simulink library "library_mtu_simulink"  (R2019a)
settings: Solver=VariableStepAuto  StartTime=0.0  StopTime=10.0  RelTol=1e-3  EnableMultiTasking=on
values from neighbouring files (symbols this model uses):
  MP = muscle_param_GM_exp    [init_muscle_exp.m]
undefined symbols (not defined in the file or in its folder): stim0
libraries: $bdroot x3
settings Model: Creator=danielhaeufle  LastModifiedBy=danielhaeufle
settings DataIOCC: LimitDataPoints=on  ReturnWorkspaceOutputs=off
settings OptimizationCC: LifeSpan=inf
settings DebuggingCC: AllowSymbolicDim=off  PregeneratedLibrarySubsystemCodeDiagnostic=none  SFUnexpectedBacktrackingDiag=warning  SFNoUnconditionalDefaultTransitionDiag=warning  SFExecutionAtInitializationDiag=none  ArithmeticOperatorsInVariantConditions=warning
settings ModelReferenceCC: PropagateSignalLabelsOutOfModel=off
settings SFSimCC: SimUseLocalCustomCode=off
settings RTWCC: RTWUseLocalCustomCode=off
settings CodeAppCC: StateflowObjectComments=on
settings GRTTargetCC: TargetLangStandard=C89/C90 (ANSI)
settings ConfigComp: CovMetricSettings=dw  CovHtmlReporting=on  CovSaveCumulativeToWorkspaceVar=on  CovSaveSingleToWorkspaceVar=on  CovExternalEMLEnable=off

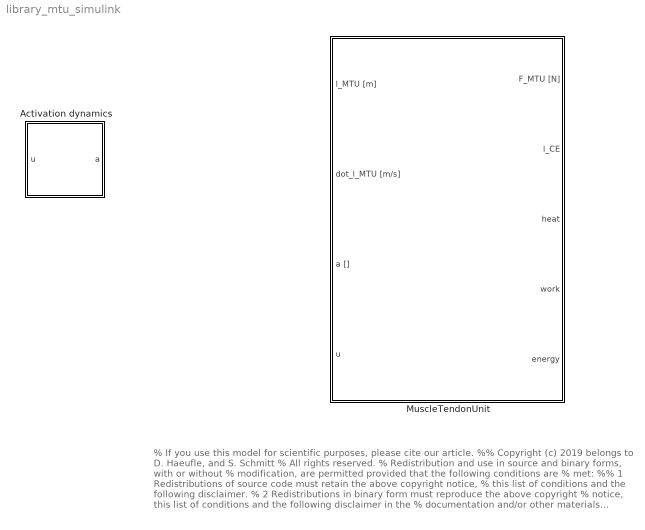
== system library_mtu_simulink ==
  note: % If you use this model for scientific purposes, please cite our article.
      | %% Copyright (c) 2019 belongs to D. Haeufle, and S. Schmitt % All rights reserved.
      | % Redistribution and use in source and binary forms, with or without
      | % modification, are permitted provided that the following conditions are
      | % met:
      | %%  1 Redistributions of source code must retain the above copyright notice,
      | %    this list of conditions and the following disclaimer.
      | %  2 Redistributions in binary form must reproduce the above copyright
      | %    notice, this list of conditions and the following disclaimer in the
      | %    documentation and/or other materials provided with the distribution.
      | %  3 Neither the name of the owner nor the names of its contributors may be
      | %    used to endorse or promote products derived from this software without
      | %    specific prior written permission.
      | %% THIS SOFTWARE IS PROVIDED BY THE COPYRIGHT HOLDERS AND CONTRIBUTORS "AS
      | % IS" AND ANY EXPRESS OR IMPLIED WARRANTIES, INCLUDING, BUT NOT LIMITED TO,
      | % THE IMPLIED WARRANTIES OF MERCHANTABILITY AND FITNESS FOR A PARTICULAR
      | % PURPOSE ARE DISCLAIMED. IN NO EVENT SHALL THE COPYRIGHT HOLDER BE LIABLE
      | % FOR ANY DIRECT, INDIRECT, INCIDENTAL, SPECIAL, EXEMPLARY, OR
      | % CONSEQUENTIAL DAMAGES (INCLUDING, BUT NOT LIMITED TO, PROCUREMENT OF
      | % SUBSTITUTE GOODS OR SERVICES; LOSS OF USE, DATA, OR PROFITS; OR BUSINESS
      | % INTERRUPTION) HOWEVER CAUSED AND ON ANY THEORY OF LIABILITY, WHETHER IN
      | % CONTRACT, STRICT LIABILITY, OR TORT (INCLUDING NEGLIGENCE OR OTHERWISE)
      | % ARISING IN ANY WAY OUT OF THE USE OF THIS SOFTWARE, EVEN IF ADVISED OF
      | % THE POSSIBILITY OF SUCH DAMAGE.
  Activation dynamics : Subsystem  mask{Mus_Param=MP(1)}
      mask prompts: Mus_Param "Muscle parameter struct"
  MuscleTendonUnit : Subsystem  mask(Muscle Tendon Complex Model){Mus_Param=MP(1)}
      mask prompts: Mus_Param "Muscle parameter struct"
      mask help: This block returns the muscle tendon complex (MTC) force based on muscle length l_MTC, contraction velocity dot_l_MTC, and activity q
      mask Help:
      | Copyright (c) 2013, D. Haeufle, M. Guenther, A. Bayer, and S. Schmitt
      | All rights reserved.
      | 
      | Redistribution and use in source and binary forms, with or without modification, are permitted provided that the following conditions are met:
      | 
      |     Redistributions of source code must retain the above copyright notice, this list of conditions and the following disclaimer.
      |     Redistributions in binary form must reproduce the above copyright notice, this list of conditions and the following disclaimer in the documentation and/or other materials provided with the distribution.
      |     Neither the name of the <ORGANIZATION> nor the names of its contributors may be used to endorse or promote products derived from this software without specific prior written permission.
      | 
      | THIS SOFTWARE IS PROVIDED BY THE COPYRIGHT HOLDERS AND CONTRIBUTORS "AS IS" AND ANY EXPRESS OR IMPLIED WARRANTIES, INCLUDING, BUT NOT LIMITED TO, THE IMPLIED WARRANTIES OF MERCHANTABILITY AND FITNESS FOR A PARTICULAR PURPOSE ARE DISCLAIMED. IN NO EVENT SHALL THE COPYRIGHT HOLDER OR CONTRIBUTORS BE LIABLE FOR ANY DIRECT, INDIRECT, INCIDENTAL, SPECIAL, EXEMPLARY, OR CONSEQUENTIAL DAMAGES (INCLUDING, BUT NOT LIMITED TO, PROCUREMENT OF SUBSTITUTE GOODS OR SERVICES; LOSS OF USE, DATA, OR PROFITS; OR BUSINESS INTERRUPTION) HOWEVER CAUSED AND ON ANY THEORY OF LIABILITY, WHETHER IN CONTRACT, STRICT LIABILITY, OR TORT (INCLUDING NEGLIGENCE OR OTHERWISE) ARISING IN ANY WAY OUT OF THE USE OF THIS SOFTWARE, EVEN IF ADVISED OF THE POSSIBILITY OF SUCH DAMAGE.
      mask Display: patch([4 4 4 4 3.5 3 2.6 2.2 2 2.2 2.6 3 3.5 4 4 4 4 7 7 7 7 7.5 8 8.4 8.8 9 8.8 8.4 8 7.5 7 7 7 7 4]/20+0.2, [0 2:17 17:-1:2 0 0]/17,[1 0 0])

== system library_mtu_simulink/Activation dynamics ==
  u : Inport
  Add1 : Sum  Inputs=-+
  Add3 : Sum
  Constant : Constant  Value=Mus_Param.act_dyn.c1
  Constant1 : Constant  Value=Mus_Param.act_dyn.c2
  Integrator : Integrator  InitialConditionSource=external  InitialCondition=stim0
  Product : Product
  Product1 : Product
  initial activity : Constant  Value=Mus_Param.a_CE_init
  a : Outport
  wires:
  u/1 -> Product1/1, Add1/2
  Integrator/1 -> Add1/1, a/1
  Product/1 -> Integrator/1
  Add1/1 -> Product/1
  initial activity/1 -> Integrator/2
  Constant/1 -> Product1/2
  Product1/1 -> Add3/1
  Add3/1 -> Product/2
  Constant1/1 -> Add3/2

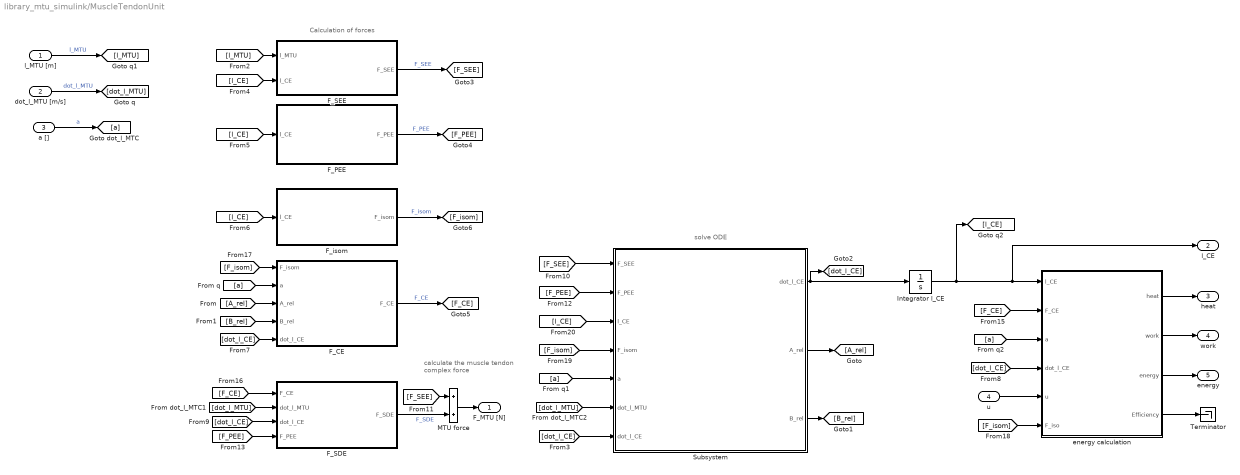
== system library_mtu_simulink/MuscleTendonUnit ==
  note: solve ODE
  note: Calculation of forces
  note: calculate the
      | muscle tendon complex
      | force
  l_MTU [m] : Inport
  dot_l_MTU [m/s] : Inport  Port=2
  a [] : Inport  Port=3
  u : Inport  Port=4
  F_CE : Subsystem
  F_PEE : Subsystem
  F_SDE : Subsystem
  F_SEE : Subsystem
  F_isom : Subsystem
  Integrator l_CE : Integrator  InitialCondition=Mus_Param.l_CE_init  ZeroCross=off
  MTU force : Sum
  Subsystem : Subsystem
  Terminator : Terminator
  energy calculation : Subsystem
  F_MTU [N] : Outport
  l_CE : Outport  Port=2
  heat : Outport  Port=3
  work : Outport  Port=4
  energy : Outport  Port=5
  wires:
  F_isom/1(F_isom) -> [F_isom]  "F_isom"
  F_PEE/1(F_PEE) -> [F_PEE]  "F_PEE"
  F_SEE/1(F_SEE) -> [F_SEE]  "F_SEE"
  F_CE/1(F_CE) -> [F_CE]  "F_CE"
  F_SDE/1(F_SDE) -> MTU force/2  "F_SDE"
  MTU force/1 -> F_MTU [N]/1
  [a] -> F_CE/2(a)
  [a] -> Subsystem/5("a ")
  [dot_l_CE] -> Subsystem/7(dot_l_CE)
  [dot_l_MTU] -> F_SDE/2(dot_l_MTU)
  Subsystem/2(A_rel) -> [A_rel]
  a []/1 -> [a]  "a"
  energy calculation/1(heat) -> heat/1
  u/1 -> energy calculation/5(u)
  energy calculation/2(work) -> work/1
  [A_rel] -> F_CE/3(A_rel)
  [B_rel] -> F_CE/4(B_rel)
  Subsystem/3(B_rel) -> [B_rel]
  Integrator l_CE/1 -> [l_CE], l_CE/1, energy calculation/1(l_CE)
  energy calculation/3(energy) -> energy/1
  Subsystem/1("dot_l_CE ") -> [dot_l_CE], Integrator l_CE/1
  l_MTU [m]/1 -> [l_MTU]  "l_MTU"
  dot_l_MTU [m/s]/1 -> [dot_l_MTU]  "dot_l_MTU"
  [l_MTU] -> F_SEE/1(l_MTU)
  [l_CE] -> F_SEE/2(l_CE)
  [l_CE] -> F_PEE/1(l_CE)
  [l_CE] -> F_isom/1(l_CE)
  [dot_l_CE] -> F_CE/5(dot_l_CE)
  [dot_l_CE] -> energy calculation/4(dot_l_CE)
  [a] -> energy calculation/3(a)
  [dot_l_CE] -> F_SDE/3(dot_l_CE)
  [F_SEE] -> Subsystem/1(F_SEE)
  [F_SEE] -> MTU force/1
  [F_PEE] -> Subsystem/2(F_PEE)
  [F_PEE] -> F_SDE/4(F_PEE)
  [F_CE] -> energy calculation/2(F_CE)
  [F_CE] -> F_SDE/1(F_CE)
  [F_isom] -> F_CE/1(F_isom)
  [F_isom] -> energy calculation/6(F_iso)
  [F_isom] -> Subsystem/4(F_isom)
  [l_CE] -> Subsystem/3(l_CE)
  [dot_l_MTU] -> Subsystem/6(dot_l_MTU)
  energy calculation/4(Efficiency) -> Terminator/1

== system library_mtu_simulink/MuscleTendonUnit/F_CE ==
  note: force of the contractile element
  F_isom : Inport
  a : Inport  Port=2
  A_rel : Inport  Port=3
  B_rel : Inport  Port=4
  dot_l_CE : Inport  Port=5
  Mux : Mux  Inputs=5
  equation for F_CE : Fcn  Expr="Mus_Param.CE.F_max * (  ( (u(1)*u(4)+u(2)) / ( 1- (u(5)/(u(3)*Mus_Param.CE.l_CEopt)) ) )-u(2) )"
  F_CE : Outport
  wires:
  a/1 -> Mux/1
  A_rel/1 -> Mux/2
  B_rel/1 -> Mux/3
  F_isom/1 -> Mux/4
  dot_l_CE/1 -> Mux/5
  equation for F_CE/1 -> F_CE/1
  Mux/1 -> equation for F_CE/1

== system library_mtu_simulink/MuscleTendonUnit/F_PEE ==
  note: Parallel elastic element force
      |
      | is only calculated if l_CE>PEE slack length
      | to avoid complex numbers with
      | non-integer exponents
  l_CE : Inport
  "F_PEE " : Subsystem
  l_PEE > slack length? : Fcn  Expr=(u>=Mus_Param.PEE.l_PEE0)
  F_PEE : Outport
  wires:
  l_CE/1 -> l_PEE > slack length?/1, "F_PEE "/1(l_PEE)
  "F_PEE "/1(Out1) -> F_PEE/1
  l_PEE > slack length?/1 -> "F_PEE "/Enable

== system library_mtu_simulink/MuscleTendonUnit/F_SDE ==
  note: force of the serial damping element
  F_CE : Inport
  dot_l_MTU : Inport  Port=2
  dot_l_CE : Inport  Port=3
  F_PEE : Inport  Port=4
  Mux : Mux
  equation for F_SDE : Fcn  Expr=Mus_Param.SDE.d_SEmax*((1-Mus_Param.SDE.R_SE)*((u(1)+u(2))/Mus_Param.CE.F_max)+Mus_Param.SDE.R_SE)*(u(3)-u(4))
  F_SDE : Outport
  wires:
  Mux/1 -> equation for F_SDE/1
  F_PEE/1 -> Mux/2
  F_CE/1 -> Mux/1
  equation for F_SDE/1 -> F_SDE/1
  dot_l_MTU/1 -> Mux/3
  dot_l_CE/1 -> Mux/4

== system library_mtu_simulink/MuscleTendonUnit/F_SEE ==
  note: MP.SEE.l_SEEnll = L_SEE (angespannt)
  note: MP.SEE.l_SEE0 = rest length of SEE in [m] (Ruhelage)
  note: Series elastic element force
  l_MTU : Inport
  l_CE : Inport  Port=2
  Add1 : Sum  Inputs=+-
  F_SEE_eq : Subsystem
  F_SEE : Outport
  wires:
  l_CE/1 -> Add1/2
  F_SEE_eq/1(F_SEE) -> F_SEE/1
  Add1/1 -> F_SEE_eq/1(l_SEE)  "l_SE"
  l_MTU/1 -> Add1/1

== system library_mtu_simulink/MuscleTendonUnit/F_isom ==
  note: isometric force-length relation
  l_CE : Inport
  Add : Sum
  ascending branch : Fcn  Expr="(Mus_Param.CE.l_CEopt>u)   *   ( exp( -( abs(  ((u/Mus_Param.CE.l_CEopt)-1)/Mus_Param.CE.DeltaW_limb_asc  ) )^Mus_Param.CE.v_CElimb_asc ) )"
  descending branch : Fcn  Expr="(Mus_Param.CE.l_CEopt<=u)   *   ( exp( -( abs(  ((u/Mus_Param.CE.l_CEopt)-1)/Mus_Param.CE.DeltaW_limb_des  ) )^Mus_Param.CE.v_CElimb_des ) )"
  F_isom : Outport
  wires:
  l_CE/1 -> descending branch/1, ascending branch/1
  Add/1 -> F_isom/1
  ascending branch/1 -> Add/2
  descending branch/1 -> Add/1

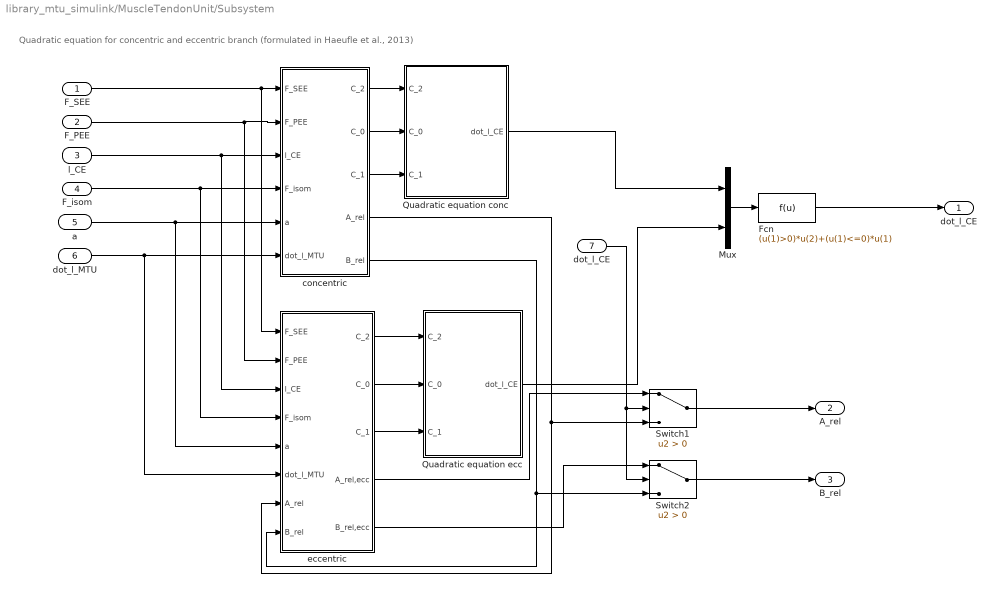
== system library_mtu_simulink/MuscleTendonUnit/Subsystem ==
  note: Quadratic equation for concentric and eccentric branch (formulated in Haeufle et al., 2013)
  F_SEE : Inport
  F_PEE : Inport  Port=2
  l_CE : Inport  Port=3
  F_isom : Inport  Port=4
  "a " : Inport  Port=5
  dot_l_MTU : Inport  Port=6
  dot_l_CE : Inport  Port=7
  Fcn : Fcn  Expr=(u(1)>0)*u(2)+(u(1)<=0)*u(1)
  Mux : Mux  Inputs=2
  Quadratic equation conc : Subsystem
  Quadratic equation ecc : Subsystem
  Switch1 : Switch  Criteria=u2 > Threshold
  Switch2 : Switch  Criteria=u2 > Threshold
  concentric : Subsystem
  eccentric : Subsystem
  "dot_l_CE " : Outport
  A_rel : Outport  Port=2
  B_rel : Outport  Port=3
  wires:
  dot_l_MTU/1 -> eccentric/6(dot_l_MTU), concentric/6(dot_l_MTU)
  F_PEE/1 -> concentric/2(F_PEE), eccentric/2(F_PEE)
  l_CE/1 -> eccentric/3(l_CE), concentric/3(l_CE)
  concentric/3("C_1 ") -> Quadratic equation conc/3(C_1)
  concentric/5(B_rel) -> Switch2/3, eccentric/8(B_rel)
  F_SEE/1 -> eccentric/1(F_SEE), concentric/1(F_SEE)
  F_isom/1 -> eccentric/4(F_isom), concentric/4(F_isom)
  "a "/1 -> eccentric/5(a), concentric/5(a)
  concentric/2("C_0 ") -> Quadratic equation conc/2(C_0)
  concentric/4(A_rel) -> Switch1/3, eccentric/7(A_rel)
  concentric/1("C_2 ") -> Quadratic equation conc/1(C_2)
  eccentric/1("C_2 ") -> Quadratic equation ecc/1(C_2)
  eccentric/2("C_0 ") -> Quadratic equation ecc/2(C_0)
  eccentric/3("C_1 ") -> Quadratic equation ecc/3(C_1)
  dot_l_CE/1 -> Switch2/2, Switch1/2
  Quadratic equation ecc/1(dot_l_CE) -> Mux/2
  Switch1/1 -> A_rel/1
  Switch2/1 -> B_rel/1
  eccentric/4(A_rel,ecc) -> Switch1/1
  eccentric/5(B_rel,ecc) -> Switch2/1
  Mux/1 -> Fcn/1
  Quadratic equation conc/1(dot_l_CE) -> Mux/1
  Fcn/1 -> "dot_l_CE "/1

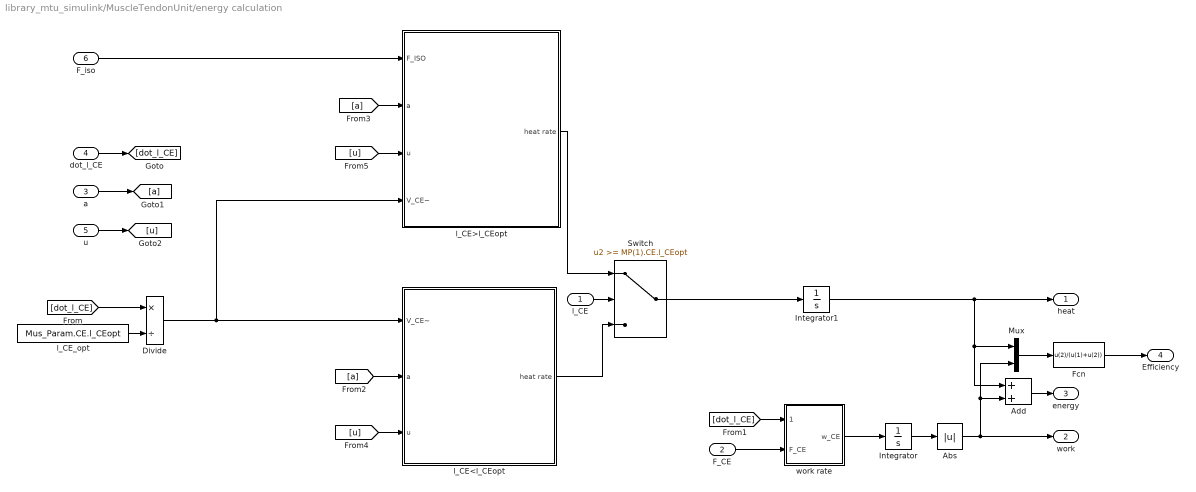
== system library_mtu_simulink/MuscleTendonUnit/energy calculation ==
  l_CE : Inport
  F_CE : Inport  Port=2
  a : Inport  Port=3
  dot_l_CE : Inport  Port=4
  u : Inport  Port=5
  F_iso : Inport  Port=6
  Abs : Abs
  Add : Sum
  Divide : Product  Inputs=*/
  Fcn : Fcn  Expr=u(2)/(u(1)+u(2))
  Integrator : Integrator
  Integrator1 : Integrator
  Mux : Mux  Inputs=2
  Switch : Switch  Threshold=MP(1).CE.l_CEopt
  l_CE<l_CEopt : Subsystem
  l_CE>l_CEopt : Subsystem
  l_CE_opt : Constant  Value=Mus_Param.CE.l_CEopt
  work rate : Subsystem
  heat : Outport
  work : Outport  Port=2
  energy : Outport  Port=3
  Efficiency : Outport  Port=4
  wires:
  Divide/1 -> l_CE>l_CEopt/4(V_CE~), l_CE<l_CEopt/1(V_CE~)
  l_CE_opt/1 -> Divide/2
  l_CE<l_CEopt/1(heat rate) -> Switch/3
  l_CE>l_CEopt/1(heat rate) -> Switch/1
  Add/1 -> energy/1
  F_iso/1 -> l_CE>l_CEopt/1(F_ISO)
  Integrator1/1 -> Mux/1, Add/1, heat/1
  F_CE/1 -> work rate/2(F_CE)
  l_CE/1 -> Switch/2
  Switch/1 -> Integrator1/1
  work rate/1(w_CE) -> Integrator/1
  Mux/1 -> Fcn/1
  Fcn/1 -> Efficiency/1
  Integrator/1 -> Abs/1
  Abs/1 -> Mux/2, Add/2, work/1
  dot_l_CE/1 -> [dot_l_CE]
  [dot_l_CE] -> Divide/1
  [dot_l_CE] -> work rate/1(dot_l_CE)
  a/1 -> [a]
  [a] -> l_CE<l_CEopt/2(a)
  [a] -> l_CE>l_CEopt/2(a)
  u/1 -> [u]
  [u] -> l_CE<l_CEopt/3(u)
  [u] -> l_CE>l_CEopt/3(u)

== system library_mtu_simulink/MuscleTendonUnit/F_PEE/F_PEE  ==
  l_PEE : Inport
  Enable : EnablePort  StatesWhenEnabling=reset
  "F_PEE " : Fcn  Expr=Mus_Param.PEE.K_PEE*(u-Mus_Param.PEE.l_PEE0)^(Mus_Param.PEE.v_PEE)
  Out1 : Outport  InitialOutput=0
  wires:
  l_PEE/1 -> "F_PEE "/1
  "F_PEE "/1 -> Out1/1

== system library_mtu_simulink/MuscleTendonUnit/F_SEE/F_SEE_eq ==
  l_SEE : Inport
  Add : Sum
  linear part : Fcn  Expr="(u>=Mus_Param.SEE.l_SEEnll)   *   (Mus_Param.SEE.DeltaF_SEE0+Mus_Param.SEE.KSEEl*(u-Mus_Param.SEE.l_SEEnll))"
  non-linear part1 : Fcn  Expr="(u>Mus_Param.SEE.l_SEE0)*(u<Mus_Param.SEE.l_SEEnll)  *  Mus_Param.SEE.KSEEnl*((u-Mus_Param.SEE.l_SEE0)^(Mus_Param.SEE.v_SEE))"
  F_SEE : Outport
  wires:
  non-linear part1/1 -> Add/2
  l_SEE/1 -> linear part/1, non-linear part1/1
  linear part/1 -> Add/1
  Add/1 -> F_SEE/1

== system library_mtu_simulink/MuscleTendonUnit/Subsystem/Quadratic equation conc ==
  note: Quadratic equation eccentric (Haeufle et al., 2013)
  C_2 : Inport
  C_0 : Inport  Port=2
  C_1 : Inport  Port=3
  Fcn1 : Fcn  Expr=(-u(3)-sqrt(u(3)^2-4*u(1)*u(2)))/(2*u(1))
  Mux : Mux  Inputs=3
  dot_l_CE : Outport
  wires:
  C_2/1 -> Mux/1
  C_0/1 -> Mux/2
  C_1/1 -> Mux/3
  Mux/1 -> Fcn1/1
  Fcn1/1 -> dot_l_CE/1

== system library_mtu_simulink/MuscleTendonUnit/Subsystem/Quadratic equation ecc ==
  note: Quadratic equation eccentric (Haeufle et al., 2013)
  C_2 : Inport
  C_0 : Inport  Port=2
  C_1 : Inport  Port=3
  Fcn1 : Fcn  Expr=(-u(3)+sqrt(u(3)^2-4*u(1)*u(2)))/(2*u(1))
  Mux : Mux  Inputs=3
  dot_l_CE : Outport
  wires:
  C_2/1 -> Mux/1
  C_0/1 -> Mux/2
  C_1/1 -> Mux/3
  Mux/1 -> Fcn1/1
  Fcn1/1 -> dot_l_CE/1

== system library_mtu_simulink/MuscleTendonUnit/Subsystem/concentric ==
  F_SEE : Inport
  F_PEE : Inport  Port=2
  l_CE : Inport  Port=3
  F_isom : Inport  Port=4
  a : Inport  Port=5
  dot_l_MTU : Inport  Port=6
  Berechnung Parameter : Subsystem
  Subsystem1 : Subsystem
  "C_2 " : Outport
  "C_0 " : Outport  Port=2
  "C_1 " : Outport  Port=3
  A_rel : Outport  Port=4
  B_rel : Outport  Port=5
  wires:
  l_CE/1 -> Subsystem1/1(l_CE)
  Subsystem1/1(A_rel) -> A_rel/1, Berechnung Parameter/5("A_rel ")
  dot_l_MTU/1 -> Berechnung Parameter/6(dot_l_MTU)
  F_isom/1 -> Berechnung Parameter/3(F_isom), Subsystem1/3(F_isom)
  F_SEE/1 -> Berechnung Parameter/1(F_SEE)
  Subsystem1/2(B_rel) -> B_rel/1, Berechnung Parameter/7(B_rel)
  Berechnung Parameter/3("C_1 ") -> "C_1 "/1
  F_PEE/1 -> Berechnung Parameter/2("F_PEE ")
  Berechnung Parameter/1("C_2 ") -> "C_2 "/1
  Berechnung Parameter/2("C_0 ") -> "C_0 "/1
  a/1 -> Subsystem1/2("q "), Berechnung Parameter/4("a ")

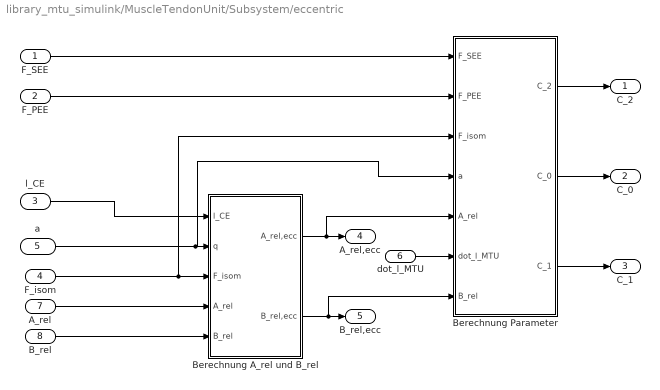
== system library_mtu_simulink/MuscleTendonUnit/Subsystem/eccentric ==
  F_SEE : Inport
  F_PEE : Inport  Port=2
  l_CE : Inport  Port=3
  F_isom : Inport  Port=4
  a : Inport  Port=5
  dot_l_MTU : Inport  Port=6
  A_rel : Inport  Port=7
  B_rel : Inport  Port=8
  Berechnung A_rel und B_rel : Subsystem
  Berechnung Parameter : Subsystem
  "C_2 " : Outport
  "C_0 " : Outport  Port=2
  "C_1 " : Outport  Port=3
  A_rel,ecc : Outport  Port=4
  B_rel,ecc : Outport  Port=5
  wires:
  l_CE/1 -> Berechnung A_rel und B_rel/1(l_CE)
  Berechnung A_rel und B_rel/1(A_rel,ecc) -> Berechnung Parameter/5("A_rel "), A_rel,ecc/1
  dot_l_MTU/1 -> Berechnung Parameter/6(dot_l_MTU)
  F_isom/1 -> Berechnung Parameter/3(F_isom), Berechnung A_rel und B_rel/3(F_isom)
  F_SEE/1 -> Berechnung Parameter/1(F_SEE)
  Berechnung A_rel und B_rel/2(B_rel,ecc) -> Berechnung Parameter/7(B_rel), B_rel,ecc/1
  Berechnung Parameter/3("C_1 ") -> "C_1 "/1
  F_PEE/1 -> Berechnung Parameter/2("F_PEE ")
  Berechnung Parameter/1("C_2 ") -> "C_2 "/1
  Berechnung Parameter/2("C_0 ") -> "C_0 "/1
  a/1 -> Berechnung Parameter/4("a "), Berechnung A_rel und B_rel/2("q ")
  A_rel/1 -> Berechnung A_rel und B_rel/4(A_rel)
  B_rel/1 -> Berechnung A_rel und B_rel/5(B_rel)

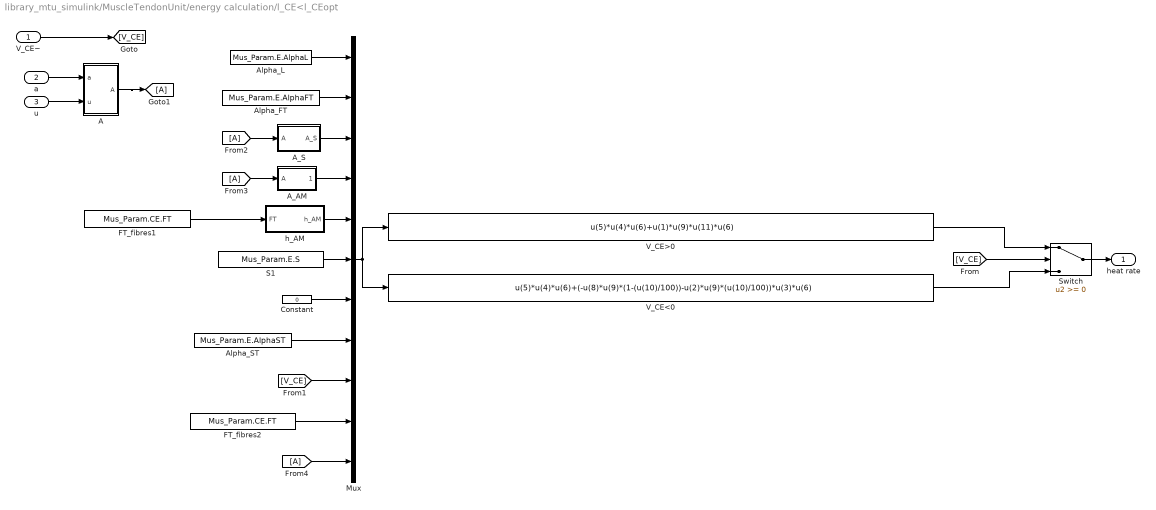
== system library_mtu_simulink/MuscleTendonUnit/energy calculation/l_CE<l_CEopt ==
  V_CE~ : Inport
  a : Inport  Port=2
  u : Inport  Port=3
  A : Subsystem
  A_AM : Subsystem
  A_S : Subsystem
  Alpha_FT : Constant  Value=Mus_Param.E.AlphaFT
  Alpha_L : Constant  Value=Mus_Param.E.AlphaL
  Alpha_ST : Constant  Value=Mus_Param.E.AlphaST
  Constant : Constant  Value=0
  FT_fibres1 : Constant  Value=Mus_Param.CE.FT
  FT_fibres2 : Constant  Value=Mus_Param.CE.FT
  Mux : Mux  Inputs=11
  S1 : Constant  Value=Mus_Param.E.S
  Switch : Switch
  V_CE<0 : Fcn  Expr=u(5)*u(4)*u(6)+(-u(8)*u(9)*(1-(u(10)/100))-u(2)*u(9)*(u(10)/100))*u(3)*u(6)
  V_CE>0 : Fcn  Expr=u(5)*u(4)*u(6)+u(1)*u(9)*u(11)*u(6)
  h_AM : Subsystem
  heat rate : Outport
  wires:
  a/1 -> A/1(a)
  u/1 -> A/2(u)
  A/1(A) -> [A]
  V_CE~/1 -> [V_CE]
  FT_fibres1/1 -> h_AM/1(FT)
  Alpha_ST/1 -> Mux/8
  Alpha_L/1 -> Mux/1
  Alpha_FT/1 -> Mux/2
  A_S/1(A_S) -> Mux/3
  A_AM/1(A_AM) -> Mux/4
  h_AM/1(h_AM) -> Mux/5
  S1/1 -> Mux/6
  Mux/1 -> V_CE<0/1, V_CE>0/1
  Switch/1 -> heat rate/1
  V_CE>0/1 -> Switch/1
  V_CE<0/1 -> Switch/3
  [V_CE] -> Switch/2
  [V_CE] -> Mux/9
  [A] -> A_S/1(A)
  [A] -> A_AM/1(A)
  [A] -> Mux/11
  Constant/1 -> Mux/7
  FT_fibres2/1 -> Mux/10

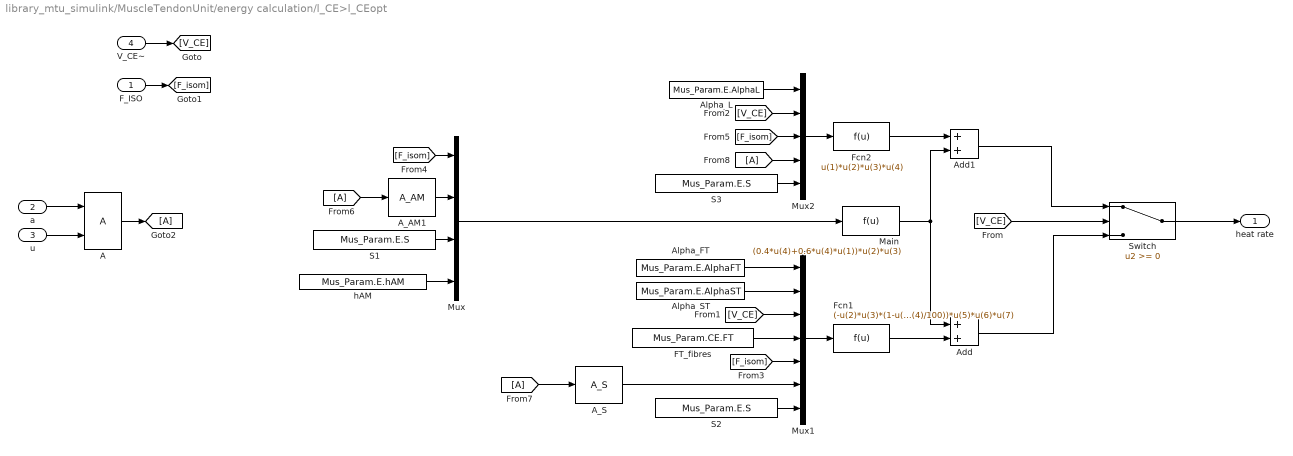
== system library_mtu_simulink/MuscleTendonUnit/energy calculation/l_CE>l_CEopt ==
  F_ISO : Inport
  a : Inport  Port=2
  u : Inport  Port=3
  V_CE~ : Inport  Port=4
  A : $bdroot/MuscleTendonUnit/energy calculation/l_CE<l_CEopt/A
  A_AM1 : $bdroot/MuscleTendonUnit/energy calculation/l_CE<l_CEopt/A_AM
  A_S : $bdroot/MuscleTendonUnit/energy calculation/l_CE<l_CEopt/A_S
  Add : Sum
  Add1 : Sum
  Alpha_FT : Constant  Value=Mus_Param.E.AlphaFT
  Alpha_L : Constant  Value=Mus_Param.E.AlphaL
  Alpha_ST : Constant  Value=Mus_Param.E.AlphaST
  FT_fibres : Constant  Value=Mus_Param.CE.FT
  Fcn1 : Fcn  Expr=(-u(2)*u(3)*(1-u(4)/100)-u(1)*u(3)*(u(4)/100))*u(5)*u(6)*u(7)
  Fcn2 : Fcn  Expr=u(1)*u(2)*u(3)*u(4)
  Main : Fcn  Expr=(0.4*u(4)+0.6*u(4)*u(1))*u(2)*u(3)
  Mux : Mux
  Mux1 : Mux  Inputs=7
  Mux2 : Mux  Inputs=5
  S1 : Constant  Value=Mus_Param.E.S
  S2 : Constant  Value=Mus_Param.E.S
  S3 : Constant  Value=Mus_Param.E.S
  Switch : Switch
  hAM : Constant  Value=Mus_Param.E.hAM
  heat rate : Outport
  wires:
  FT_fibres/1 -> Mux1/4
  a/1 -> A/1
  u/1 -> A/2
  A_AM1/1 -> Mux/2
  Mux/1 -> Main/1
  Alpha_FT/1 -> Mux1/1
  Alpha_ST/1 -> Mux1/2
  A_S/1 -> Mux1/6
  Mux1/1 -> Fcn1/1
  Alpha_L/1 -> Mux2/1
  Mux2/1 -> Fcn2/1
  Switch/1 -> heat rate/1
  Main/1 -> Add1/2, Add/1
  Fcn2/1 -> Add1/1
  hAM/1 -> Mux/4
  Add1/1 -> Switch/1
  Add/1 -> Switch/3
  V_CE~/1 -> [V_CE]
  [V_CE] -> Switch/2
  [V_CE] -> Mux1/3
  [V_CE] -> Mux2/2
  F_ISO/1 -> [F_isom]
  [F_isom] -> Mux1/5
  [F_isom] -> Mux/1
  [F_isom] -> Mux2/3
  S1/1 -> Mux/3
  S2/1 -> Mux1/7
  S3/1 -> Mux2/5
  A/1 -> [A]
  [A] -> A_AM1/1
  [A] -> A_S/1
  [A] -> Mux2/4
  Fcn1/1 -> Add/2

== system library_mtu_simulink/MuscleTendonUnit/energy calculation/work rate ==
  dot_l_CE : Inport
  F_CE : Inport  Port=2
  Divide1 : Product  Inputs=*/
  Gain : Gain  Gain=-1
  PCSA : Constant  Value=Mus_Param.E.PCSA
  Product1 : Product
  Product2 : Product  Inputs=3
  l_CE_opt1 : Constant  Value=Mus_Param.CE.l_CEopt
  p_density : Constant  Value=Mus_Param.E.muscle_density
  w_CE : Outport
  wires:
  Product1/1 -> Divide1/1
  dot_l_CE/1 -> Product1/2
  F_CE/1 -> Product1/1
  Divide1/1 -> Gain/1
  Gain/1 -> w_CE/1
  p_density/1 -> Product2/1
  PCSA/1 -> Product2/2
  l_CE_opt1/1 -> Product2/3
  Product2/1 -> Divide1/2  "muscle mass"

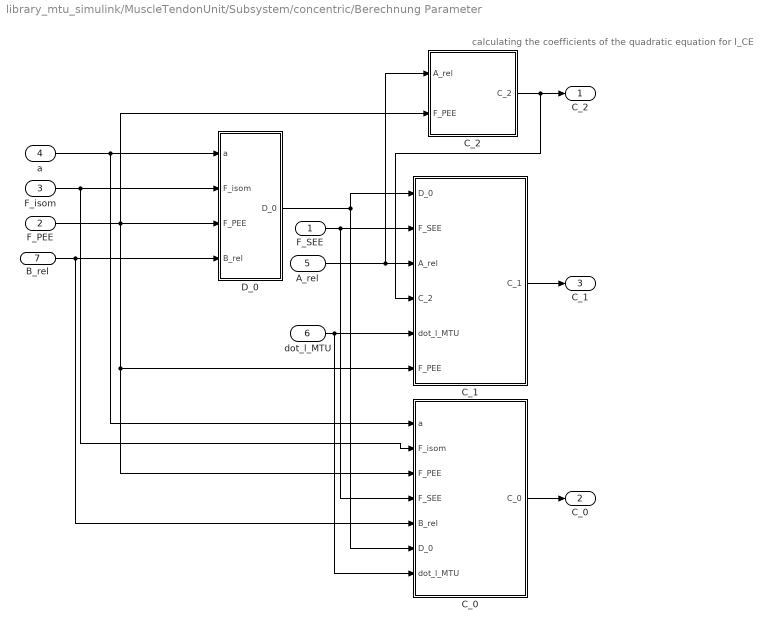
== system library_mtu_simulink/MuscleTendonUnit/Subsystem/concentric/Berechnung Parameter ==
  note: calculating the coefficients of the quadratic equation for l_CE
  F_SEE : Inport
  "F_PEE " : Inport  Port=2
  F_isom : Inport  Port=3
  "a " : Inport  Port=4
  "A_rel " : Inport  Port=5
  dot_l_MTU : Inport  Port=6
  B_rel : Inport  Port=7
  C_0 : Subsystem
  C_1 : Subsystem
  C_2 : Subsystem
  D_0 : Subsystem
  "C_2 " : Outport
  "C_0 " : Outport  Port=2
  "C_1 " : Outport  Port=3
  wires:
  "a "/1 -> C_0/1(a), D_0/1(a)
  C_0/1(C_0) -> "C_0 "/1
  C_1/1(C_1) -> "C_1 "/1
  dot_l_MTU/1 -> C_0/7(dot_l_MTU), C_1/5(dot_l_MTU)
  F_isom/1 -> C_0/2(F_isom), D_0/2(F_isom)
  C_2/1(C_2) -> C_1/4(C_2), "C_2 "/1
  D_0/1(D_0) -> C_1/1(D_0), C_0/6(D_0)
  "A_rel "/1 -> C_1/3(A_rel), C_2/1(A_rel)
  F_SEE/1 -> C_0/4(F_SEE), C_1/2(F_SEE)
  "F_PEE "/1 -> C_0/3(F_PEE), C_1/6(F_PEE), C_2/2(F_PEE), D_0/3(F_PEE)
  B_rel/1 -> C_0/5(B_rel), D_0/4(B_rel)

== system library_mtu_simulink/MuscleTendonUnit/Subsystem/concentric/Subsystem1 ==
  note: Parameter of Hills' hyperbola
  l_CE : Inport
  "q " : Inport  Port=2
  F_isom : Inport  Port=3
  Arel : Subsystem
  Brel : Fcn  Expr=Mus_Param.CE.B_rel0*1*1/7*(3+4*u)
  A_rel : Outport
  B_rel : Outport  Port=2
  wires:
  Brel/1 -> B_rel/1
  "q "/1 -> Brel/1, Arel/1(q)
  F_isom/1 -> Arel/3(F_isom)
  Arel/1(A_rel) -> A_rel/1
  l_CE/1 -> Arel/2(l_CE)

== system library_mtu_simulink/MuscleTendonUnit/Subsystem/eccentric/Berechnung A_rel und B_rel ==
  note: Parameter of Hills' hyperbola
  l_CE : Inport
  "q " : Inport  Port=2
  F_isom : Inport  Port=3
  A_rel : Inport  Port=4
  B_rel : Inport  Port=5
  Arel,ecc : Subsystem
  Brel,ecc : Subsystem
  A_rel,ecc : Outport
  B_rel,ecc : Outport  Port=2
  wires:
  "q "/1 -> Brel,ecc/1(q), Arel,ecc/1(q)
  F_isom/1 -> Brel,ecc/4(F_isom), Arel,ecc/3(F_isom)
  Arel,ecc/1("A_rel,ecc ") -> A_rel,ecc/1
  l_CE/1 -> Arel,ecc/2(l_CE)
  Brel,ecc/1(B_rel,ecc) -> B_rel,ecc/1
  A_rel/1 -> Brel,ecc/2("A_rel ")
  B_rel/1 -> Brel,ecc/3("B_rel ")

== system library_mtu_simulink/MuscleTendonUnit/Subsystem/eccentric/Berechnung Parameter ==
  note: calculating the coefficients of the quadratic equation for l_CE
  F_SEE : Inport
  "F_PEE " : Inport  Port=2
  F_isom : Inport  Port=3
  "a " : Inport  Port=4
  "A_rel " : Inport  Port=5
  dot_l_MTU : Inport  Port=6
  B_rel : Inport  Port=7
  C_0 : Subsystem
  C_1 : Subsystem
  C_2 : Subsystem
  D_0 : Subsystem
  "C_2 " : Outport
  "C_0 " : Outport  Port=2
  "C_1 " : Outport  Port=3
  wires:
  "a "/1 -> C_0/1(a), D_0/1(a)
  C_0/1(C_0) -> "C_0 "/1
  C_1/1(C_1) -> "C_1 "/1
  dot_l_MTU/1 -> C_0/7(dot_l_MTU), C_1/5(dot_l_MTU)
  F_isom/1 -> C_0/2(F_isom), D_0/2(F_isom)
  C_2/1(C_2) -> C_1/4(C_2), "C_2 "/1
  D_0/1(D_0) -> C_1/1(D_0), C_0/6(D_0)
  "A_rel "/1 -> C_1/3(A_rel), C_2/1(A_rel)
  F_SEE/1 -> C_0/4(F_SEE), C_1/2(F_SEE)
  "F_PEE "/1 -> C_0/3(F_PEE), C_1/6(F_PEE), C_2/2(F_PEE), D_0/3(F_PEE)
  B_rel/1 -> C_0/5(B_rel), D_0/4(B_rel)

== system library_mtu_simulink/MuscleTendonUnit/energy calculation/l_CE<l_CEopt/A ==
  a : Inport
  u : Inport  Port=2
  Add : Sum
  Product : Product
  Switch2 : Switch  Criteria=u2 > Threshold  Threshold=[MP(1).a_CE_init]
  const : Constant  Value=0.5
  A : Outport
  wires:
  Add/1 -> Product/1
  const/1 -> Product/2
  Switch2/1 -> A/1
  Product/1 -> Switch2/3
  a/1 -> Add/2
  u/1 -> Add/1, Switch2/2, Switch2/1

== system library_mtu_simulink/MuscleTendonUnit/energy calculation/l_CE<l_CEopt/A_AM ==
  A : Inport
  Constant : Constant  Value=0.6
  Math Function : Math  Operator=pow  SaturateOnIntegerOverflow=on
  A_AM : Outport
  wires:
  Math Function/1 -> A_AM/1
  A/1 -> Math Function/1
  Constant/1 -> Math Function/2

== system library_mtu_simulink/MuscleTendonUnit/energy calculation/l_CE<l_CEopt/A_S ==
  A : Inport
  Constant : Constant  Value=2.0
  Math Function : Math  Operator=pow  SaturateOnIntegerOverflow=on
  A_S : Outport
  wires:
  A/1 -> Math Function/1
  Constant/1 -> Math Function/2
  Math Function/1 -> A_S/1

== system library_mtu_simulink/MuscleTendonUnit/energy calculation/l_CE<l_CEopt/h_AM ==
  FT : Inport
  Add : Sum
  Product : Product
  const : Constant  Value=1.28
  const2 : Constant  Value=25
  h_AM : Outport
  wires:
  const/1 -> Product/2
  Product/1 -> Add/1
  Add/1 -> h_AM/1
  const2/1 -> Add/2
  FT/1 -> Product/1

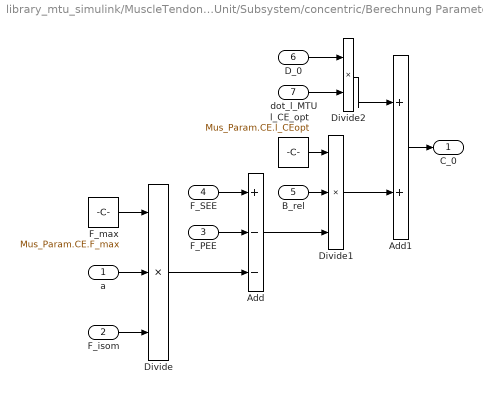
== system library_mtu_simulink/MuscleTendonUnit/Subsystem/concentric/Berechnung Parameter/C_0 ==
  a : Inport
  F_isom : Inport  Port=2
  F_PEE : Inport  Port=3
  F_SEE : Inport  Port=4
  B_rel : Inport  Port=5
  D_0 : Inport  Port=6
  dot_l_MTU : Inport  Port=7
  Add : Sum  Inputs=+--
  Add1 : Sum
  Divide : Product  Inputs=***
  Divide1 : Product  Inputs=***
  Divide2 : Product  Inputs=**
  F_max : Constant  Value=Mus_Param.CE.F_max
  l_CE_opt : Constant  Value=Mus_Param.CE.l_CEopt
  C_0 : Outport
  wires:
  F_max/1 -> Divide/1
  a/1 -> Divide/2
  F_isom/1 -> Divide/3
  Divide/1 -> Add/3
  F_PEE/1 -> Add/2
  F_SEE/1 -> Add/1
  Add/1 -> Divide1/3
  B_rel/1 -> Divide1/2
  Divide2/1 -> Add1/1
  Add1/1 -> C_0/1
  D_0/1 -> Divide2/1
  dot_l_MTU/1 -> Divide2/2
  l_CE_opt/1 -> Divide1/1
  Divide1/1 -> Add1/2

== system library_mtu_simulink/MuscleTendonUnit/Subsystem/concentric/Berechnung Parameter/C_1 ==
  D_0 : Inport
  F_SEE : Inport  Port=2
  A_rel : Inport  Port=3
  C_2 : Inport  Port=4
  dot_l_MTU : Inport  Port=5
  F_PEE : Inport  Port=6
  Add : Sum  Inputs=---+-
  Divide : Product  Inputs=**
  Divide1 : Product  Inputs=**
  F_max : Constant  Value=Mus_Param.CE.F_max
  C_1 : Outport
  wires:
  F_max/1 -> Divide/1
  A_rel/1 -> Divide/2
  Divide/1 -> Add/5
  Divide1/1 -> Add/1
  C_2/1 -> Divide1/1
  dot_l_MTU/1 -> Divide1/2
  D_0/1 -> Add/2
  F_SEE/1 -> Add/3
  F_PEE/1 -> Add/4
  Add/1 -> C_1/1

== system library_mtu_simulink/MuscleTendonUnit/Subsystem/concentric/Berechnung Parameter/C_2 ==
  A_rel : Inport
  F_PEE : Inport  Port=2
  1 : Constant
  Add : Sum  Inputs=+-
  Add1 : Sum  Inputs=+-
  Add2 : Sum  Inputs=+-
  Divide : Product  Inputs=*/
  Divide1 : Product  Inputs=**
  Divide2 : Product  Inputs=**
  F_max : Constant  Value=Mus_Param.CE.F_max
  R_SE : Constant  Value=Mus_Param.SDE.R_SE
  R_SE1 : Constant  Value=Mus_Param.SDE.R_SE
  d_SEmax : Constant  Value=Mus_Param.SDE.d_SEmax
  C_2 : Outport
  wires:
  A_rel/1 -> Add/1
  Divide/1 -> Add/2
  F_PEE/1 -> Divide/1
  F_max/1 -> Divide/2
  Add/1 -> Divide1/1
  Add1/1 -> Divide1/2
  1/1 -> Add1/1
  R_SE/1 -> Add1/2
  Divide1/1 -> Add2/2
  R_SE1/1 -> Add2/1
  Add2/1 -> Divide2/1
  d_SEmax/1 -> Divide2/2
  Divide2/1 -> C_2/1

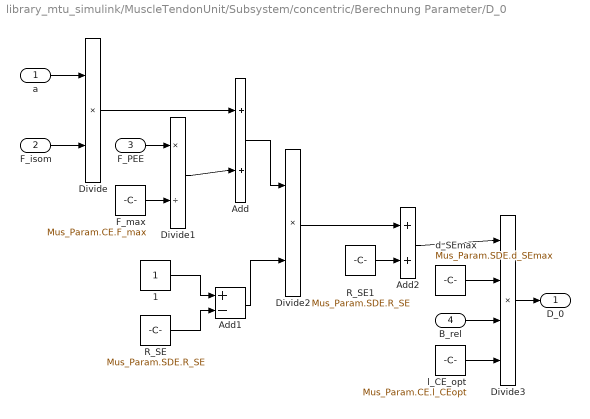
== system library_mtu_simulink/MuscleTendonUnit/Subsystem/concentric/Berechnung Parameter/D_0 ==
  a : Inport
  F_isom : Inport  Port=2
  F_PEE : Inport  Port=3
  B_rel : Inport  Port=4
  1 : Constant
  Add : Sum
  Add1 : Sum  Inputs=+-
  Add2 : Sum
  Divide : Product  Inputs=**
  Divide1 : Product  Inputs=*/
  Divide2 : Product  Inputs=**
  Divide3 : Product  Inputs=****
  F_max : Constant  Value=Mus_Param.CE.F_max
  R_SE : Constant  Value=Mus_Param.SDE.R_SE
  R_SE1 : Constant  Value=Mus_Param.SDE.R_SE
  d_SEmax : Constant  Value=Mus_Param.SDE.d_SEmax
  l_CE_opt : Constant  Value=Mus_Param.CE.l_CEopt
  D_0 : Outport
  wires:
  a/1 -> Divide/1
  F_isom/1 -> Divide/2
  Divide/1 -> Add/1
  F_PEE/1 -> Divide1/1
  F_max/1 -> Divide1/2
  Divide1/1 -> Add/2
  Add/1 -> Divide2/1
  1/1 -> Add1/1
  R_SE/1 -> Add1/2
  Add1/1 -> Divide2/2
  Divide2/1 -> Add2/1
  R_SE1/1 -> Add2/2
  Add2/1 -> Divide3/1
  d_SEmax/1 -> Divide3/2
  l_CE_opt/1 -> Divide3/4
  B_rel/1 -> Divide3/3
  Divide3/1 -> D_0/1

== system library_mtu_simulink/MuscleTendonUnit/Subsystem/concentric/Subsystem1/Arel ==
  q : Inport
  l_CE : Inport  Port=2
  F_isom : Inport  Port=3
  Arel : Fcn  Expr=( 1.0*(u(2)<Mus_Param.CE.l_CEopt) + u(3)*(u(2)>=Mus_Param.CE.l_CEopt) )*Mus_Param.CE.A_rel0*1/4*(1+3*u(1))
  Mux : Mux  Inputs=3
  A_rel : Outport
  wires:
  Mux/1 -> Arel/1
  F_isom/1 -> Mux/3
  l_CE/1 -> Mux/2
  q/1 -> Mux/1
  Arel/1 -> A_rel/1

== system library_mtu_simulink/MuscleTendonUnit/Subsystem/eccentric/Berechnung A_rel und B_rel/Arel,ecc ==
  q : Inport
  l_CE : Inport  Port=2
  F_isom : Inport  Port=3
  Arel : Fcn  Expr=-Mus_Param.CE.F_eccentric*u(1)*u(3)
  Mux : Mux  Inputs=3
  "A_rel,ecc " : Outport
  wires:
  Mux/1 -> Arel/1
  F_isom/1 -> Mux/3
  l_CE/1 -> Mux/2
  q/1 -> Mux/1
  Arel/1 -> "A_rel,ecc "/1

== system library_mtu_simulink/MuscleTendonUnit/Subsystem/eccentric/Berechnung A_rel und B_rel/Brel,ecc ==
  q : Inport
  "A_rel " : Inport  Port=2
  "B_rel " : Inport  Port=3
  F_isom : Inport  Port=4
  Brel : Fcn  Expr=u(1)*u(2)*(1-Mus_Param.CE.F_eccentric)/(u(1)*u(2)+u(3))*u(4)/Mus_Param.CE.S_eccentric
  Mux : Mux
  B_rel,ecc : Outport
  wires:
  Brel/1 -> B_rel,ecc/1
  q/1 -> Mux/1
  F_isom/1 -> Mux/2
  "A_rel "/1 -> Mux/3
  "B_rel "/1 -> Mux/4
  Mux/1 -> Brel/1

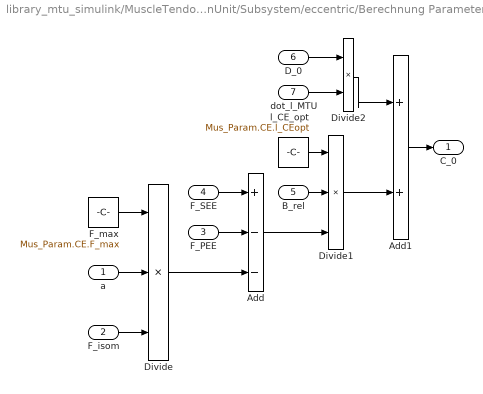
== system library_mtu_simulink/MuscleTendonUnit/Subsystem/eccentric/Berechnung Parameter/C_0 ==
  a : Inport
  F_isom : Inport  Port=2
  F_PEE : Inport  Port=3
  F_SEE : Inport  Port=4
  B_rel : Inport  Port=5
  D_0 : Inport  Port=6
  dot_l_MTU : Inport  Port=7
  Add : Sum  Inputs=+--
  Add1 : Sum
  Divide : Product  Inputs=***
  Divide1 : Product  Inputs=***
  Divide2 : Product  Inputs=**
  F_max : Constant  Value=Mus_Param.CE.F_max
  l_CE_opt : Constant  Value=Mus_Param.CE.l_CEopt
  C_0 : Outport
  wires:
  F_max/1 -> Divide/1
  a/1 -> Divide/2
  F_isom/1 -> Divide/3
  Divide/1 -> Add/3
  F_PEE/1 -> Add/2
  F_SEE/1 -> Add/1
  Add/1 -> Divide1/3
  B_rel/1 -> Divide1/2
  Divide2/1 -> Add1/1
  Add1/1 -> C_0/1
  D_0/1 -> Divide2/1
  dot_l_MTU/1 -> Divide2/2
  l_CE_opt/1 -> Divide1/1
  Divide1/1 -> Add1/2

== system library_mtu_simulink/MuscleTendonUnit/Subsystem/eccentric/Berechnung Parameter/C_1 ==
  D_0 : Inport
  F_SEE : Inport  Port=2
  A_rel : Inport  Port=3
  C_2 : Inport  Port=4
  dot_l_MTU : Inport  Port=5
  F_PEE : Inport  Port=6
  Add : Sum  Inputs=---+-
  Divide : Product  Inputs=**
  Divide1 : Product  Inputs=**
  F_max : Constant  Value=Mus_Param.CE.F_max
  C_1 : Outport
  wires:
  F_max/1 -> Divide/1
  A_rel/1 -> Divide/2
  Divide/1 -> Add/5
  Divide1/1 -> Add/1
  C_2/1 -> Divide1/1
  dot_l_MTU/1 -> Divide1/2
  D_0/1 -> Add/2
  F_SEE/1 -> Add/3
  F_PEE/1 -> Add/4
  Add/1 -> C_1/1

== system library_mtu_simulink/MuscleTendonUnit/Subsystem/eccentric/Berechnung Parameter/C_2 ==
  A_rel : Inport
  F_PEE : Inport  Port=2
  1 : Constant
  Add : Sum  Inputs=+-
  Add1 : Sum  Inputs=+-
  Add2 : Sum  Inputs=+-
  Divide : Product  Inputs=*/
  Divide1 : Product  Inputs=**
  Divide2 : Product  Inputs=**
  F_max : Constant  Value=Mus_Param.CE.F_max
  R_SE : Constant  Value=Mus_Param.SDE.R_SE
  R_SE1 : Constant  Value=Mus_Param.SDE.R_SE
  d_SEmax : Constant  Value=Mus_Param.SDE.d_SEmax
  C_2 : Outport
  wires:
  A_rel/1 -> Add/1
  Divide/1 -> Add/2
  F_PEE/1 -> Divide/1
  F_max/1 -> Divide/2
  Add/1 -> Divide1/1
  Add1/1 -> Divide1/2
  1/1 -> Add1/1
  R_SE/1 -> Add1/2
  Divide1/1 -> Add2/2
  R_SE1/1 -> Add2/1
  Add2/1 -> Divide2/1
  d_SEmax/1 -> Divide2/2
  Divide2/1 -> C_2/1

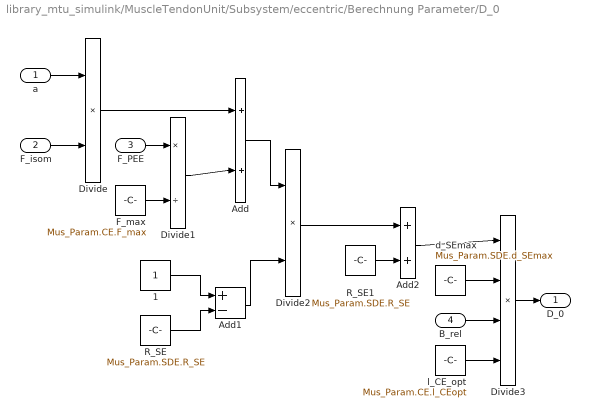
== system library_mtu_simulink/MuscleTendonUnit/Subsystem/eccentric/Berechnung Parameter/D_0 ==
  a : Inport
  F_isom : Inport  Port=2
  F_PEE : Inport  Port=3
  B_rel : Inport  Port=4
  1 : Constant
  Add : Sum
  Add1 : Sum  Inputs=+-
  Add2 : Sum
  Divide : Product  Inputs=**
  Divide1 : Product  Inputs=*/
  Divide2 : Product  Inputs=**
  Divide3 : Product  Inputs=****
  F_max : Constant  Value=Mus_Param.CE.F_max
  R_SE : Constant  Value=Mus_Param.SDE.R_SE
  R_SE1 : Constant  Value=Mus_Param.SDE.R_SE
  d_SEmax : Constant  Value=Mus_Param.SDE.d_SEmax
  l_CE_opt : Constant  Value=Mus_Param.CE.l_CEopt
  D_0 : Outport
  wires:
  a/1 -> Divide/1
  F_isom/1 -> Divide/2
  Divide/1 -> Add/1
  F_PEE/1 -> Divide1/1
  F_max/1 -> Divide1/2
  Divide1/1 -> Add/2
  Add/1 -> Divide2/1
  1/1 -> Add1/1
  R_SE/1 -> Add1/2
  Add1/1 -> Divide2/2
  Divide2/1 -> Add2/1
  R_SE1/1 -> Add2/2
  Add2/1 -> Divide3/1
  d_SEmax/1 -> Divide3/2
  l_CE_opt/1 -> Divide3/4
  B_rel/1 -> Divide3/3
  Divide3/1 -> D_0/1
